simulink model "Switching_losses"  (R2015a)
settings: Solver=ode45  StartTime=0.0  StopTime=10.0  RelTol=1e-3
undefined symbols (not defined in the file or in its folder): Vdc
settings Model: Creator=Caner  LastModifiedBy=Caner

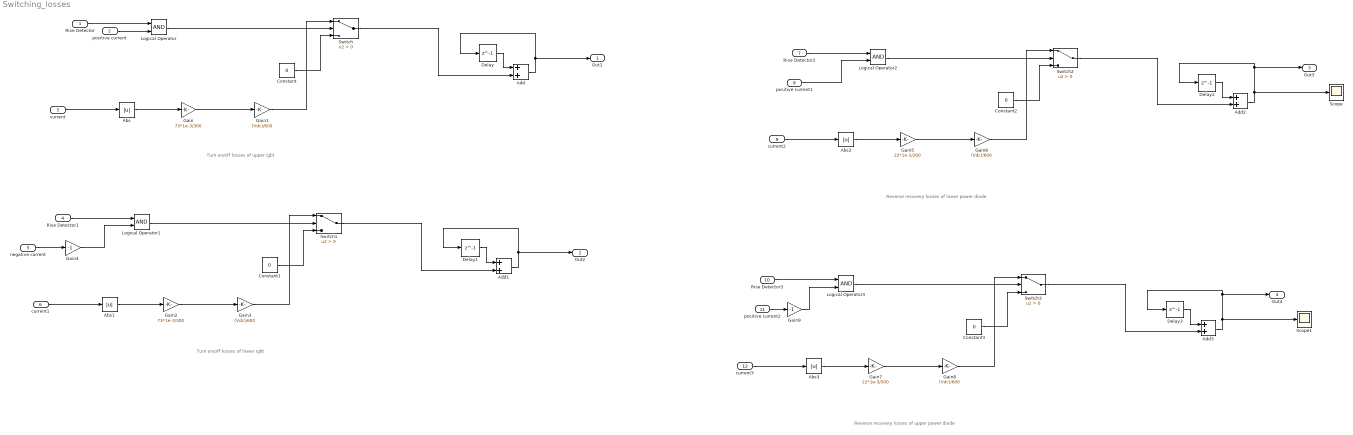
== system Switching_losses ==
  note: Reverse recovery losses of lower power diode
  note: Turn on/off losses of lower igbt
  note: Turn on/off losses of upper igbt
  note: Reverse recovery losses of upper power diode
  Rise Detector : Inport
  positive current : Inport  Port=2
  current : Inport  Port=3
  Rise Detector1 : Inport  Port=4
  negative current : Inport  Port=5
  current1 : Inport  Port=6
  Rise Detector2 : Inport  Port=7
  positive current1 : Inport  Port=8
  current2 : Inport  Port=9
  Rise Detector3 : Inport  Port=10
  positive current2 : Inport  Port=11
  current3 : Inport  Port=12
  Abs{,1..3} (4 alike) : Abs
  Add{,1..3} (4 alike) : Sum
  Constant{,1..3} (4 alike) : Constant  Value=0
  Delay{,1..3} (4 alike) : Delay  DelayLength=1  InitialCondition=0
  Gain : Gain  Gain=73*1e-3/300
  Gain{1,3,6,8} (4 alike) : Gain  Gain=(Vdc)/600
  Gain2 : Gain  Gain=73*1e-3/300
  Gain4 : Gain  Gain=-1
  Gain5 : Gain  Gain=22*1e-3/300
  Gain7 : Gain  Gain=22*1e-3/300
  Gain9 : Gain  Gain=-1
  Logical Operator{,1..3} (4 alike) : Logic  AllPortsSameDT=off  OutDataTypeStr=boolean
  Scope : Scope
  Scope1 : Scope
  Switch{,1..3} (4 alike) : Switch  Criteria=u2 > Threshold
  Out1 : Outport
  Out2 : Outport  Port=2
  Out3 : Outport  Port=3
  Out4 : Outport  Port=4
  wires:
  Rise Detector/1 -> Logical Operator/1
  positive current/1 -> Logical Operator/2
  Logical Operator/1 -> Switch/2
  current/1 -> Abs/1
  Abs/1 -> Gain/1
  Gain/1 -> Gain1/1
  Gain1/1 -> Switch/1
  Constant/1 -> Switch/3
  Add/1 -> Delay/1, Out1/1
  Delay/1 -> Add/1
  Switch/1 -> Add/2
  Rise Detector1/1 -> Logical Operator1/1
  negative current/1 -> Gain4/1
  Logical Operator1/1 -> Switch1/2
  current1/1 -> Abs1/1
  Abs1/1 -> Gain2/1
  Gain2/1 -> Gain3/1
  Gain3/1 -> Switch1/1
  Constant1/1 -> Switch1/3
  Add1/1 -> Delay1/1, Out2/1
  Delay1/1 -> Add1/1
  Switch1/1 -> Add1/2
  Gain4/1 -> Logical Operator1/2
  Rise Detector2/1 -> Logical Operator2/1
  positive current1/1 -> Logical Operator2/2
  Logical Operator2/1 -> Switch2/2
  current2/1 -> Abs2/1
  Abs2/1 -> Gain5/1
  Gain5/1 -> Gain6/1
  Gain6/1 -> Switch2/1
  Constant2/1 -> Switch2/3
  Add2/1 -> Scope/1, Delay2/1, Out3/1
  Delay2/1 -> Add2/1
  Switch2/1 -> Add2/2
  Rise Detector3/1 -> Logical Operator3/1
  positive current2/1 -> Gain9/1
  Logical Operator3/1 -> Switch3/2
  current3/1 -> Abs3/1
  Abs3/1 -> Gain7/1
  Gain7/1 -> Gain8/1
  Gain8/1 -> Switch3/1
  Constant3/1 -> Switch3/3
  Add3/1 -> Scope1/1, Delay3/1, Out4/1
  Delay3/1 -> Add3/1
  Switch3/1 -> Add3/2
  Gain9/1 -> Logical Operator3/2
